simulink model "1"  (R2024b)
settings: Solver=FixedStepDiscrete  StartTime=0.0  StopTime=25  FixedStep=1e-5  RelTol=1e-3
libraries: simulink x1
settings Model: Creator=86195  LastModifiedBy=86195

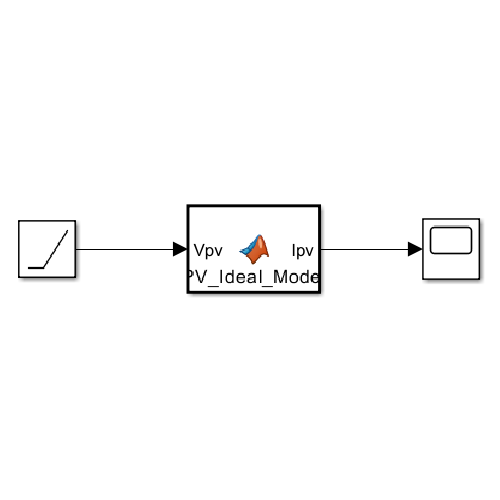
[thumbnail: Simulink's stored preview of the top-level diagram]
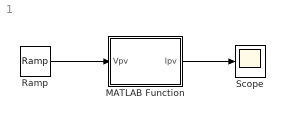
== system 1 ==
  MATLAB Function : MATLAB Function  TreatAsAtomicUnit=on
  Ramp : simulink/Sources/Ramp  slope=1  start=0  InitialOutput=0
  Scope : Scope
  wires:
  Ramp/1 -> MATLAB Function/1(Vpv)
  MATLAB Function/1(Ipv) -> Scope/1

== matlab function 1/MATLAB Function ==
  data: Vpv input; Ipv output
function Ipv = PV_Ideal_Model(Vpv)
%%光伏电池理想模型的搭建
%%常数量
k = 1.38e-23;%玻尔兹曼常数
q = 1.60e-19;%单位电荷量
%%给定参数
T = 25+273;%光伏电池温度
A = 0.97359;%二极管的品质因数
Iph  = 3.8;%光生电流
Is = 2.4515e-10;%二极管反向饱和电流
Ns = 36;%光伏组件串联光伏单体数量
%%公式
Vt = k*T/q;%光伏电池热电压
Vpv = Vpv/Ns;%计算每个串联光伏单体的电压
Id = Is*(exp(Vpv/(A*Vt))-1);%二极管电流，其中二极管电压Vd等于光伏电池电压
Ipv = Iph - Id;
